simulink model "Six_DoF_LQR"  (R2020a)
settings: Solver=VariableStepAuto  StartTime=0.0  StopTime=P.t_end  RelTol=1e-3
InitFcn:
  | drone_param
StartFcn:
  | drone_param
values from neighbouring files (symbols this model uses):
  P = drone_linearization(P)    [drone_param.m]
undefined symbols (not defined in the file or in its folder): drawDrone
ContinueFcn:
  | FT2frfl
settings Model: Creator=sadam  LastModifiedBy=sadam
settings DataIOCC: ReturnWorkspaceOutputs=off
settings DebuggingCC: ArithmeticOperatorsInVariantConditions=warning
settings SFSimCC: SimUseLocalCustomCode=off  CustomCodeUndefinedFunction=UseInterfaceOnly
settings RTWCC: RTWUseLocalCustomCode=off

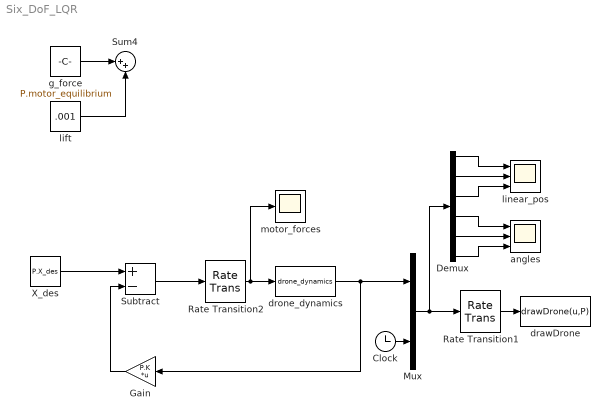
== system Six_DoF_LQR ==
  Clock : Clock
  Demux : Demux  Outputs=6
  Gain : Gain  Gain=P.K  Multiplication=Matrix(K*u)
  Mux : Mux  Inputs=2
  Rate Transition1 : RateTransition  OutPortSampleTime=P.t_plot
  Rate Transition2 : RateTransition  OutPortSampleTime=P.Ts
  Subtract : Sum  Inputs=+-
  Sum4 : Sum  Inputs=|++
  X_des : Constant  Value=P.X_des
  angles : Scope  NumInputPorts=3
  drawDrone : MATLABFcn  MATLABFcn=drawDrone(u,P)  OutputDimensions=0
  drone_dynamics : S-Function  FunctionName=drone_dynamics  Parameters=P  SFunctionDeploymentMode=off  EnableBusSupport=off
  g_force : Constant  Value=P.motor_equilibrium
  lift : Constant  Value=.001
  linear_pos : Scope  NumInputPorts=3
  motor_forces : Scope
  wires:
  Rate Transition1/1 -> drawDrone/1
  drone_dynamics/1 -> Gain/1, Mux/1
  Clock/1 -> Mux/2
  Mux/1 -> Demux/1, Rate Transition1/1
  Rate Transition2/1 -> motor_forces/1, drone_dynamics/1
  g_force/1 -> Sum4/1
  lift/1 -> Sum4/2
  Demux/1 -> linear_pos/1
  Demux/2 -> linear_pos/2
  Demux/3 -> linear_pos/3
  Demux/4 -> angles/1
  Demux/5 -> angles/2
  Demux/6 -> angles/3
  Subtract/1 -> Rate Transition2/1
  Gain/1 -> Subtract/2
  X_des/1 -> Subtract/1
